simulink library "TestSequence"  (R2014b)
settings: Solver=ode45  StartTime=0.0  StopTime=10.0  RelTol=1e-3
undefined symbols (not defined in the file): sigbuilder_block
settings Model: Creator=dan  LastModifiedBy=dan

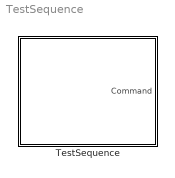
== system TestSequence ==
  TestSequence : Subsystem

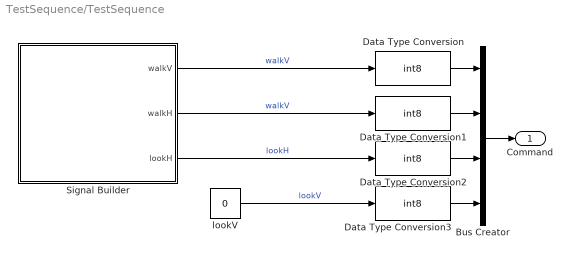
== system TestSequence/TestSequence ==
  Bus Creator : BusCreator  OutDataTypeStr=Bus: Command
      settings: InheritFromInputs=off
  Data Type Conversion{,1..3} (4 alike) : DataTypeConversion  OutDataTypeStr=int8
  Signal Builder : Subsystem  Tag=STV Subsys  LoadFcn=sigbuilder_block('load');  StartFcn=sigbuilder_block('start');  StopFcn=sigbuilder_block('stop');  ClipboardFcn=sigbuilder_block('clipboard');  mask(Sigbuilder block){}
      mask help: Simulink:masks:SigbuilderBlock_MD
      mask init:
      | if ~strcmp(get_param(bdroot(gcbh),'SimulationStatus'),'stopped') tuvar = sigbuilder_block('maskInit'); end
      settings: CopyFcn=sigbuilder_block('copy');  DeleteFcn=sigbuilder_block('delete');  ModelCloseFcn=sigbuilder_block('modelClose');  PreSaveFcn=sigbuilder_block('preSave');  PauseFcn=sigbuilder_block('pause');  ContinueFcn=sigbuilder_block('continue');  NameChangeFcn=sigbuilder_block('namechange');  OpenFcn=sigbuilder_block('open',[437.6 199.2 550.4 400 ]);  CloseFcn=sigbuilder_block('close');
      mask Display: plot(0, 0, 100, 100,[2, 2, 32, 32, 2], [68, 8, 8, 68, 68],[32, 2], [38, 38], [32, 19, 2],[53, 60, 44], [32, 17, 17, 2],[16, 16, 31, 31]);txt = getActiveGroup(gcbh);text(2, 100, txt,'verticalAlignment', 'top');
  lookV : Constant  Value=0
  Command : Outport
  wires:
  Signal Builder/3(lookH) -> Data Type Conversion2/1  "lookH"
  lookV/1 -> Data Type Conversion3/1  "lookV"
  Signal Builder/2(walkH) -> Data Type Conversion1/1  "walkV"
  Signal Builder/1(walkV) -> Data Type Conversion/1  "walkV"
  Bus Creator/1 -> Command/1
  Data Type Conversion/1 -> Bus Creator/1
  Data Type Conversion1/1 -> Bus Creator/2
  Data Type Conversion2/1 -> Bus Creator/3
  Data Type Conversion3/1 -> Bus Creator/4

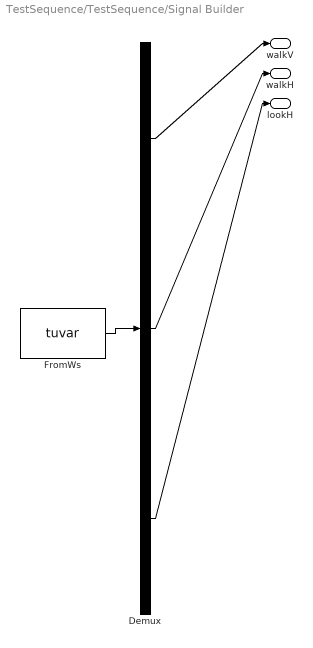
== system TestSequence/TestSequence/Signal Builder ==
  Demux : Demux  Tag=STV Demux  Outputs=3
  FromWs : FromWorkspace  Tag=STV FromWs  VariableName=tuvar  SampleTime=0
      SigBuilderData=|
      | common.afterFinalStr = 'Extrapolate'
      | common.sampleTime = 0
      | dataSet.timeRange = [0 100]
      | dataSet.name = 'Group 1'
      | sbobj.Groups.Name = 'Group 1'
      | sbobj.Groups.Signals(1).Name = 'walkV'
      | sbobj.Groups.Signals(1).XData = [0 5 20 40 50 70 80 100]
      | sbobj.Groups.Signals(1).YData = [0 8 8 50 50 20 10 0]
      | sbobj.Groups.Signals(2).Name = 'walkH'
      | sbobj.Groups.Signals(2).XData = [0 34 50 70 80 100]
      | sbobj.Groups.Signals(2).YData = [0 0 30 30 0 0]
      | sbobj.Groups.Signals(3).Name = 'lookH'
      | sbobj.Groups.Signals(3).XData = [0 2 10 20 20 40 40 50 50 60 60 100]
      | sbobj.Groups.Signals(3).YData = [0 0 0 0 15 30 0 0 -40 -40 0 10]
      | sbobj.Groups.TimeRange = [0 100]
  walkV : Outport  Tag=STV Outport
  walkH : Outport  Tag=STV Outport  Port=2
  lookH : Outport  Tag=STV Outport  Port=3
  wires:
  FromWs/1 -> Demux/1
  Demux/1 -> walkV/1
  Demux/2 -> walkH/1
  Demux/3 -> lookH/1
